simulink model "adm_pcie_9h7_dts_dual_4x100g_dsp_8b_1ant"  (R2019a)
settings: Solver=VariableStepAuto  StartTime=0.0  StopTime=10.0  RelTol=1e-3
undefined symbols (not defined in the file): datetime, fft_stages, posixtime
libraries: xbsIndex_r4 x17321, casper_library_misc x181, xps_library x11, casper_library_delays x8, casper_library_sources x8, casper_library_reorder x5, casper_library_scopes x4
(part 1 of 187)
settings Model: Creator=jackh  LastModifiedBy=mybur
settings Model: ModifiedComment=|
  | jackh -- Thu Feb 02 09:09:38 2023 -- Version 1.265
  | 
  | as compiled
settings Model: ModifiedHistory=|
  | jackh -- Thu Feb 02 09:09:38 2023 -- Version 1.265
  | 
  | as compiled
  | 
  | jackh -- Thu Feb 02 09:09:38 2023 -- Version 1.265
  | 
  | as compiled
  | 
  | jackh -- Wed Feb 01 20:29:00 2023 -- Version 1.264
  | 
  | Mitigate control change relating to 100G auto-shutoff which
  | prevents core from ever being manually disabled.
  | 
  | jackh -- Wed Jan 25 18:35:33 2023 -- Version 1.263
  | compiled 13.9
  | 
  | jackh -- Tue Jan 24 18:58:34 2023 -- Version 1.262
  | 
  | Increase non-fractional delay slope bits from 0 to 5,
  | allowing firmware-side delay extrapolation to run up to
  | 2^5 ADC samples
  | 
  | jackh -- Fri Jan 13 09:42:33 2023 -- Version 1.261
  | 
  | add options for DTS-error-induced auto 100G cutoff
  | 
  | jackh -- Thu Jan 12 13:56:07 2023 -- Version 1.260
  | 
  | Add automated 100GbE output halting on timing error detection
  | 
  | jackh -- Tue Nov 29 08:46:28 2022 -- Version 1.259
  | 
  | compiled
  | 
  | jackh -- Mon Nov 28 13:45:10 2022 -- Version 1.258
  | 
  | jackh -- Mon Nov 28 13:30:45 2022 -- Version 1.257
  | 
  | jackh -- Mon Nov 28 13:16:52 2022 -- Version 1.256
  | 
  | jackh -- Mon Nov 28 13:05:40 2022 -- Version 1.255
  | 
  | jackh -- Mon Nov 28 13:04:31 2022 -- Version 1.254
  | 
  | Bugfix -- negative fractional delays
  | 
  | jackh -- Wed Nov 23 08:43:33 2022 -- Version 1.253
  | 
  | as compiled
  | 
  | 
  | jackh -- Tue Nov 22 14:50:06 2022 -- Version 1.252
  | 
  | Rework LO precision.
  | - Make phase step register Fix45_44
  | - Allow periodic reloading
  | 
  | jackh -- Wed Nov 09 19:28:54 2022 -- Version 1.251
  | 
  | compiled
  | 
  | jackh -- Tue Nov 08 11:16:07 2022 -- Version 1.250
  | 
  | byteflip on pipeline 1 second 100G port
  | 
  | jackh -- Tue Nov 08 11:14:32 2022 -- Version 1.249
  | 
  | 13.7 -- dual 100G output
  | 
  | jackh -- Fri Nov 04 13:05:36 2022 -- Version 1.248
  | 
  | v13.7 -- use both 100G ports
  | 
  | jackh -- Mon Oct 10 10:09:12 2022 -- Version 1.247
  | 
  | as compiled
  | 
  | jackh -- Sun Oct 09 20:21:09 2022 -- Version 1.246
  | 
  | duplicate changes from LO shifter 0 for 1,2,3
  | 
  | jackh -- Sat Oct 08 20:23:11 2022 -- Version 1.245
  | as compiled
  | 
  | jackh -- Sat Oct 08 10:43:03 2022 -- Version 1.244
  | 
  | bugfix 2. Sync/data timing skew in phase rotate block
  | 
  | jackh -- Thu Oct 06 21:33:25 2022 -- Version 1.243
  | 
  | jackh -- Thu Oct 06 11:23:24 2022 -- Version 1.242
  | 
  | bugfix 1 -- timed sync in LO control should drive
  | reset of phase accumulators
  | 
  | jackh -- Thu Oct 06 10:04:46 2022 -- Version 1.241
  | 
  | compiled
  | 
  | jackh -- Wed Oct 05 14:02:44 2022 -- Version 1.240
  | 
  | v13.6
  | 
  | Add load time control for LO shift.
  | Use load time consistently through LO shift / coarse delay / phase rotate
  | 
  | jackh -- Wed Oct 05 08:55:34 2022 -- Version 1.239
  | 
  | compiled v13.5
  | 
  | jackh -- Tue Oct 04 17:52:52 2022 -- Version 1.238
  | 
  | v13.5
  | 
  | Make delay in delay tracking block signed
  | 
  | jackh -- Fri Sep 23 15:25:54 2022 -- Version 1.237
  | 
  | as compiled
  | 
  | jackh -- Thu Sep 22 10:47:01 2022 -- Version 1.236
  | 
  | Bugfix 5
  | Only allow syncs on TT multiples of 2^14 (probably 2^13 would
  | be sufficient -- this is the packetizer granularity)
  | Add reset logic to reorder (which has weird reorder-orders)
  | so that it only syncs off the first pulse after a reset
  | 
  | jackh -- Thu Sep 15 17:12:54 2022 -- Version 1.235
  | 
  | jackh -- Thu Sep 15 14:00:24 2022 -- Version 1.234
  | 
  | 13.4 bugfix 4 -- fix timing on TT load
  | 
  | jackh -- Wed Aug 24 08:02:53 2022 -- Version 1.233
  | 
  | compiled
  | 
  | jackh -- Tue Aug 23 14:04:43 2022 -- Version 1.232
  | 
  | v13.4 bugfix3 -- reduce data latency in DTS snapshot (cast) to balance sync
  | 
  | jackh -- Tue Aug 23 12:45:19 2022 -- Version 1.231
  | 
  | bugfix 2 -- recompile with oldest sample in DTS MSB.
  | Delay data relative to sync at DTS output so sync precedes by 1 clock
  | 
  | jackh -- Thu Aug 18 20:38:32 2022 -- Version 1.230
  | 
  | v13.4 bugfix 1
  | Rebuild with DTS buffer fixes
  | 
  | jackh -- Thu Aug 04 11:53:58 2022 -- Version 1.229
  | 
  | as compiled
  | 
  | jackh -- Wed Aug 03 18:39:00 2022 -- Version 1.228
  | 
  | v13.4 -- add post quant TVG which is a counter with spectrum number
  | 
  | jackh -- Wed Aug 03 12:22:54 2022 -- Version 1.227
  | 
  | as compiled
  | 
  | jackh -- Tue Aug 02 16:59:19 2022 -- Version 1.226
  | 
  | v13.3.3
  | 
  | Make LO offset input accept signed values
  | 
  | jackh -- Thu Jul 14 12:25:27 2022 -- Version 1.225
  | v13.3.2
  | 
  | change sine/cos lookup tables to 18-bit depth
  | 
  | jackh -- Fri Jul 08 12:09:48 2022 -- Version 1.224
  | 
  | jackh -- Fri Jul 08 11:59:21 2022 -- Version 1.223
  | 
  | 13.3.1
  | 
  | Make LO shift phase register 32_29
  | 
  | jackh -- Tue Jul 05 14:22:39 2022 -- Version 1.222
  | 
  | 13.2.4
  | 
  | Add 100G output snapshots and stats counters
  | 
  | jackh -- Fri Jun 17 09:21:46 2022 -- Version 1.221
  | 
  | Make PR template file relative. Increment fw revision
  | 
  | jackh -- Fri May 20 08:03:37 2022 -- Version 1.220
  | 
  | jackh -- Thu May 19 16:47:03 2022 -- Version 1.219
  | 
  | jackh -- Thu May 19 16:07:36 2022 -- Version 1.218
  | 
  | 13.2.2
  | 
  | Increase coarse delay to 512 samples
  | 
  | jackh -- Thu May 19 15:48:23 2022 -- Version 1.217
  | 
  | pipeline time offset
  | 
  | jackh -- Thu May 19 15:45:17 2022 -- Version 1.216
  | 
  | v13.2.1
  | 
  | Add aux time measurement
  | 
  | jackh -- Tue May 03 22:22:24 2022 -- Version 1.215
  | 
  | jackh -- Tue May 03 12:52:13 2022 -- Version 1.214
  | 
  | 13.2.0.1
  | 
  | - Fix FFT syncout period (now infinite)
  | - Add max_delay register to delay subsystem
  | 
  | jackh -- Tue May 03 11:06:51 2022 -- Version 1.213
  | 
  | v13.2 (should have been 13) as compiled
  | 
  | jackh -- Mon May 02 12:19:53 2022 -- Version 1.212
  | 
  | jackh -- Mon May 02 12:13:43 2022 -- Version 1.211
  | 
  | jackh -- Mon May 02 12:03:22 2022 -- Version 1.210
  | 
  | Move to 1MHz channels (2048-chan PFB; 1024 sent chans)
  | Incorporate FFT descramble mlib_devel fix
  | 
  | jackh -- Thu Apr 07 10:41:20 2022 -- Version 1.209
  | 
  | compiled
  | 
  | jackh -- Wed Apr 06 17:17:38 2022 -- Version 1.208
  | 
  | Bugfix 1
  | 
  | - Change LO offset so real part os cosine mixer (so mixing with DC does nothing)
  | - Fix cross-corr conjugation
  | - Fix cross corr acc_len computation
  | 
  | jackh -- Thu Mar 24 11:16:10 2022 -- Version 1.207
  | 
  | jackh -- Wed Mar 23 15:55:29 2022 -- Version 1.206
  | 
  | v12.2 Add sine wave generators to both pipelines.
  | Default to no added sine wave.
  | 
  | jackh -- Wed Mar 23 15:38:55 2022 -- Version 1.205
  | 
  | jackh -- Wed Mar 23 15:24:07 2022 -- Version 1.204
  | 
  | delay match sine generation and data streams
  | 
  | jackh -- Wed Mar 23 15:22:28 2022 -- Version 1.203
  | 
  | jackh -- Wed Mar 23 15:14:26 2022 -- Version 1.202
  | 
  | Add additive sinewave TVG
  | 
  | jackh -- Wed Mar 23 15:12:01 2022 -- Version 1.201
  | 
  | jackh -- Tue Mar 08 10:23:22 2022 -- Version 1.200
  | 
  | jackh -- Mon Mar 07 17:18:28 2022 -- Version 1.199
  | 
  | jackh -- Mon Mar 07 17:10:55 2022 -- Version 1.198
  | 
  | jackh -- Mon Mar 07 16:45:17 2022 -- Version 1.197
  | 
  | jackh -- Mon Mar 07 16:37:10 2022 -- Version 1.196
  | 
  | Add Corr block.
  | Allows examination of post-quantization signals, and
  | to cross correlate different IFs (useful for testing
  | in internal noisegen mode)
  | 
  | jackh -- Mon Mar 07 16:13:50 2022 -- Version 1.195
  | 
  | PFB band select reorder depth fix
  | 
  | jackh -- Thu Mar 03 13:08:01 2022 -- Version 1.194
  | 
  | jackh -- Tue Mar 01 20:34:16 2022 -- Version 1.193
  | 
  | jackh -- Tue Mar 01 17:19:43 2022 -- Version 1.192
  | 
  | jackh -- Tue Mar 01 17:10:04 2022 -- Version 1.191
  | 
  | jackh -- Tue Mar 01 16:55:54 2022 -- Version 1.190
  | 
  | jackh -- Tue Mar 01 16:45:57 2022 -- Version 1.189
  | 
  | jackh -- Tue Mar 01 15:57:56 2022 -- Version 1.188
  | 
  | jackh -- Tue Mar 01 15:49:45 2022 -- Version 1.187
  | 
  | jackh -- Tue Mar 01 15:22:14 2022 -- Version 1.186
  | 
  | jackh -- Mon Feb 28 13:26:19 2022 -- Version 1.185
  | 
  | jackh -- Mon Feb 28 13:08:19 2022 -- Version 1.184
  | 
  | jackh -- Sat Feb 26 14:41:54 2022 -- Version 1.183
  | 
  | jackh -- Fri Feb 25 18:46:11 2022 -- Version 1.182
  | 
  | jackh -- Fri Feb 25 18:45:03 2022 -- Version 1.181
  | 
  | jackh -- Thu Feb 24 15:51:36 2022 -- Version 1.180
  | 
  | update noisegen casting (just take MSBs)
  | 
  | jackh -- Thu Feb 24 15:08:58 2022 -- Version 1.179
  | 
  | v12
  | 
  | jackh -- Thu Feb 24 15:06:46 2022 -- Version 1.178
  | 
  | Move to 4x100G template
  | 
  | 
  | jackh -- Thu Feb 24 15:02:10 2022 -- Version 1.177
  | 
  | jackh -- Wed Feb 09 19:02:50 2022 -- Version 1.176
  | 
  | jackh -- Wed Feb 09 10:59:16 2022 -- Version 1.175
  | 
  | Try _again_ to fix timestamp issue.
  | This time the fix was actually simulated, and seems to work.
  | 
  | jackh -- Wed Feb 09 10:58:22 2022 -- Version 1.174
  | 
  | jackh -- Wed Feb 09 10:34:47 2022 -- Version 1.173
  | 
  | jackh -- Tue Feb 08 22:13:18 2022 -- Version 1.172
  | 
  | Change autocorr pipelining to fix timing errors
  | 
  | jackh -- Tue Feb 08 11:22:49 2022 -- Version 1.171
  | 
  | Try (again) to fix MCNT offset issue.
  | This time just propagate the time_step_bit lower MCNT counter
  | bits through to the header.
  | 
  | jackh -- Tue Feb 08 08:36:48 2022 -- Version 1.170
  | 
  | jackh -- Mon Feb 07 16:56:49 2022 -- Version 1.169
  | 
  | jackh -- Mon Feb 07 16:34:15 2022 -- Version 1.168
  | 
  | jackh -- Mon Feb 07 16:26:49 2022 -- Version 1.167
  | 
  | jackh -- Mon Feb 07 12:47:03 2022 -- Version 1.166
  | 
  | jackh -- Mon Feb 07 12:32:35 2022 -- Version 1.165
  | 
  | Add TT sync register, storing the time of the last sync
  | 
  | jackh -- Mon Feb 07 12:23:30 2022 -- Version 1.164
  | 
  | increment bugfix to 11.0.0.2
  | 
  | 
  | jackh -- Mon Feb 07 12:22:16 2022 -- Version 1.163
  | 
  | Propagate LSBs of sync time to packet headers
  | 
  | jackh -- Sat Feb 05 22:32:38 2022 -- Version 1.162
  | 
  | jackh -- Sat Feb 05 18:43:37 2022 -- Version 1.161
  | 
  | v11
  | More changes to reorder.
  | Process ADC data at 8 (not 12) bit resolution
  | Use URAM via black-box imports for coarse delay and big channel reorder
  | 
  | jackh -- Sat Feb 05 18:36:04 2022 -- Version 1.160
  | 
  | jackh -- Sat Feb 05 17:38:40 2022 -- Version 1.159
  | 
  | jackh -- Sat Feb 05 17:24:29 2022 -- Version 1.158
  | 
  | jackh -- Sat Feb 05 17:22:21 2022 -- Version 1.157
  | 
  | jackh -- Fri Feb 04 17:40:07 2022 -- Version 1.156
  | 
  | jackh -- Fri Feb 04 12:37:39 2022 -- Version 1.155
  | 
  | 64 times per packet
  | 
  | 
  | jackh -- Thu Feb 03 21:55:46 2022 -- Version 1.154
  | 
  | as compiled
  | 
  | 
  | jackh -- Thu Feb 03 14:45:04 2022 -- Version 1.153
  | 
  | jackh -- Thu Feb 03 14:28:02 2022 -- Version 1.152
  | 
  | jackh -- Thu Feb 03 13:59:18 2022 -- Version 1.151
  | 
  | jackh -- Thu Feb 03 11:15:21 2022 -- Version 1.150
  | 
  | jackh -- Wed Feb 02 16:47:47 2022 -- Version 1.149
  | 
  | jackh -- Wed Feb 02 16:40:11 2022 -- Version 1.148
  | 
  | Fix incorrect final transpose in reorder block
  | 
  | jackh -- Wed Feb 02 16:16:13 2022 -- Version 1.147
  | 
  | v8. Add channel reordering
  | 
  | Not actually necessary for 8-bit mode, but will
  | facilitate testing which is necessary for 3-bit mode
  | 
  | jackh -- Wed Feb 02 10:37:50 2022 -- Version 1.146
  | 
  | 7.0.1
  | 
  | Change coarse delay bram latency to 3 (hopefully will fix small timing fail)
  | 
  | jackh -- Wed Feb 02 10:34:03 2022 -- Version 1.145
  | 
  | jackh -- Tue Feb 01 14:52:02 2022 -- Version 1.144
  | 
  | Don't use ultraRAM for coarse delay (but we should!)
  | because it breaks sysgen. Sigh.
  | 
  | jackh -- Tue Feb 01 14:27:12 2022 -- Version 1.143
  | 
  | jackh -- Tue Feb 01 14:18:24 2022 -- Version 1.142
  | 
  | v7. Add noisegen / coarse delay
  | 
  | jackh -- Tue Feb 01 14:12:26 2022 -- Version 1.141
  | 
  | jackh -- Tue Feb 01 14:09:37 2022 -- Version 1.140
  | 
  | jackh -- Tue Feb 01 11:46:40 2022 -- Version 1.139
  | 
  | jackh -- Tue Feb 01 11:12:13 2022 -- Version 1.138
  | 
  | Add noise gen
  | 
  | jackh -- Tue Feb 01 11:01:17 2022 -- Version 1.137
  | 
  | v6.1 Harmonize input ordering convention by flipping
  | inputs so "input 0" is MSBs of data
  | 
  | jackh -- Tue Feb 01 10:38:57 2022 -- Version 1.136
  | 
  | jackh -- Mon Jan 31 13:11:04 2022 -- Version 1.135
  | 
  | jackh -- Mon Jan 31 12:33:38 2022 -- Version 1.134
  | 
  | jackh -- Mon Jan 31 12:25:15 2022 -- Version 1.133
  | 
  | jackh -- Fri Jan 28 17:22:49 2022 -- Version 1.132
  | 
  | jackh -- Fri Jan 28 17:16:19 2022 -- Version 1.131
  | 
  | jackh -- Fri Jan 28 17:06:25 2022 -- Version 1.130
  | 
  | v6.0 Add input bitstats / simulation mux
  | 
  | jackh -- Fri Jan 28 17:02:52 2022 -- Version 1.129
  | 
  | jackh -- Fri Jan 28 16:59:39 2022 -- Version 1.128
  | 
  | jackh -- Fri Jan 28 16:55:40 2022 -- Version 1.127
  | 
  | jackh -- Fri Jan 28 16:17:24 2022 -- Version 1.126
  | 
  | v5.0.2 Fix potential (but unliekly) issue with sync arm coinciding
  | with sync pulse
  | 
  | 
  | jackh -- Fri Jan 28 16:01:17 2022 -- Version 1.125
  | 
  | Attempt to fix DTS alignment unreliability (control signal CDC issue in mlib_devel)
  | 
  | jackh -- Fri Jan 28 12:51:42 2022 -- Version 1.124
  | 
  | as compiled
  | 
  | jackh -- Thu Jan 27 16:47:33 2022 -- Version 1.123
  | 
  | v5.0
  | 
  | Add sync gen logic
  | 
  | jackh -- Thu Jan 27 11:25:49 2022 -- Version 1.122
  | 
  | v4.1 Add index interval error counter
  | 
  | jackh -- Thu Jan 27 11:22:02 2022 -- Version 1.121
  | 
  | Make index 50ms -- add not-locked counter
  | 
  | 
  | jackh -- Thu Jan 27 10:32:00 2022 -- Version 1.120
  | 
  | Recompile using raw "index" pulse. Add index snapshots
  | 
  | jackh -- Wed Jan 26 15:06:47 2022 -- Version 1.119
  | 
  | jackh -- Wed Jan 26 13:46:28 2022 -- Version 1.118
  | 
  | jackh -- Wed Jan 26 13:04:56 2022 -- Version 1.117
  | 
  | jackh -- Tue Jan 25 18:32:15 2022 -- Version 1.116
  | 
  | Add index (10ms pulse?) count logic
  | 
  | jackh -- Tue Jan 25 18:31:36 2022 -- Version 1.115
  | 
  | jackh -- Tue Jan 25 11:48:12 2022 -- Version 1.114
  | 
  | jackh -- Tue Jan 25 11:41:44 2022 -- Version 1.113
  | 
  | jackh -- Tue Jan 25 11:38:37 2022 -- Version 1.112
  | 
  | Readd autocorr (needed behavioural complex mults)
  | 
  | jackh -- Mon Jan 24 20:49:54 2022 -- Version 1.111
  | 
  | comment out autocorr (causing compile fails)
  | 
  | jackh -- Mon Jan 24 20:10:36 2022 -- Version 1.110
  | 
  | jackh -- Mon Jan 24 19:58:33 2022 -- Version 1.109
  | 
  | jackh -- Mon Jan 24 19:53:28 2022 -- Version 1.108
  | 
  | autocorr floating point error fixes
  | 
  | 
  | jackh -- Mon Jan 24 19:51:34 2022 -- Version 1.107
  | 
  | jackh -- Mon Jan 24 18:28:31 2022 -- Version 1.106
  | 
  | jackh -- Mon Jan 24 18:27:12 2022 -- Version 1.105
  | 
  | Add autocorr (to pipeline 0)
  | 
  | jackh -- Mon Jan 24 18:15:24 2022 -- Version 1.104
  | 
  | Add EQTVG
  | 
  | jackh -- Mon Jan 24 13:19:54 2022 -- Version 1.103
settings DataIOCC: ReturnWorkspaceOutputs=off
settings DebuggingCC: PregeneratedLibrarySubsystemCodeDiagnostic=none  ArithmeticOperatorsInVariantConditions=warning
settings SFSimCC: SimUseLocalCustomCode=off
settings RTWCC: RTWUseLocalCustomCode=off

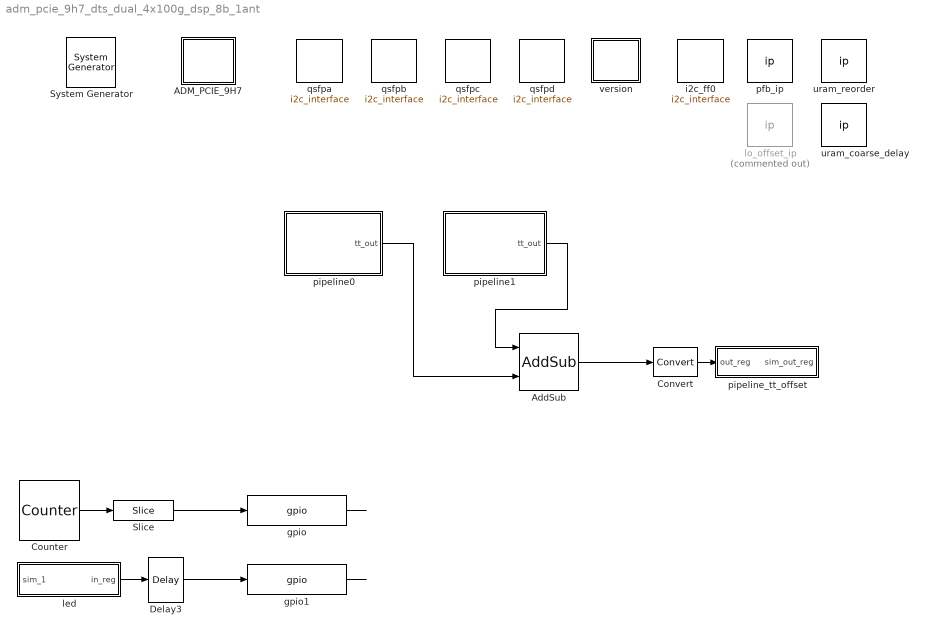
== system adm_pcie_9h7_dts_dual_4x100g_dsp_8b_1ant ==
  " System Generator" : xbsIndex_r4/ System Generator  Tag=genX  xilinxfamily=virtexuplusHBM  part=xcvu37p  speed=-2-e  package=fsvh2892  synthesis_tool=XST  clock_wrapper=Clock Enables  directory=/home/jackh/src/vla-dev/firmware/adm_pcie_9h7_dts_dual_4x100g_dsp_8b/sysgen  proj_type=Vivado  Synth_file=Vivado Synthesis Defaults  Impl_file=Vivado Implementation Defaults  testbench=off  simulink_period=1  sysclk_period=3.9062  dcm_input_clock_period=10  incr_netlist=off  trim_vbits=Everywhere in SubSystem  dbl_ovrd=According to Block Masks  core_generation=According to Block Masks  run_coregen=off  deprecated_control=off  eval_field=0  block_type=sysgen
  ADM_PCIE_9H7 : Subsystem  Tag=xps:xsg  mask(xsg core config){hw_sys=ADM_PCIE_9H7:xcvu37p, clk_src=dts_clk, clk_rate=256, use_microblaze=off, use_pr=on, pr_template=[fileparts(which(bdroot)) '/pr_templates/adm_pcie_9h7_dts_dual_4x100g_pr_template-no-ip.xpr.zip'], sample_period=1, synthesis_tool=XST}
      mask prompts: hw_sys "Hardware Platform"; clk_src "User IP Clock source"; clk_rate "User IP Clock Rate (MHz)"; use_microblaze "Use Microblaze controller?"; use_pr "Use PCIe Partial Reconfiguration"; sample_period "Sample Period"; synthesis_tool "Synthesis Tool:"
      mask help:
      | The XSG Core Config block is used to configure the System Generator design
      | for the casper_xps toolflow. Settings here are used to configure the
      | Xilinx System Generator block parameters automatically, and control toolflow
      | script  execution. It needs to be at the top level of all designs being compiled
      | with the casper_xps toolflow.
      mask init:
      | xps_xsg_adm_pcie_9h7_conf_mask;
      mask Help: eval('xlWeb([getenv(''MLIB_ROOT''), ''\doc\html\sys_xsg_core_config\sys_xsg_core_config.html''])')
      mask TypeOptions hw_sys: ADM_PCIE_9H7:xcvu37p
      mask TypeOptions clk_src: sys_clk | dts_clk
      mask TypeOptions synthesis_tool: Leonardo Spectrum | Synplify | Synplify Pro | XST
      mask Display: fprintf(['ADM\nPCIE_9H7']);
  AddSub : xbsIndex_r4/AddSub  mode=Subtraction  use_carryin=off  use_carryout=off  en=off  latency=3  precision=Full  arith_type=Unsigned  n_bits=16  bin_pt=14  quantization=Truncate  overflow=Wrap  use_behavioral_HDL=off  hw_selection=Fabric  pipelined=on  dbl_ovrd=off  block_type=addsub
  Convert : xbsIndex_r4/Convert  gui_display_data_type=Fixed-point  arith_type="Signed  (2's comp)"  n_bits=32  bin_pt=0  float_type=Single  exp_bits=8  fraction_bits=24  quantization=Truncate  overflow=Wrap  en=off  latency=1  pipeline=off  dbl_ovrd=off  block_type=convert
  Counter : xbsIndex_r4/Counter  cnt_type=Free Running  cnt_to=Inf  operation=Up  start_count=0  cnt_by_val=1  arith_type=Unsigned  n_bits=27  bin_pt=0  load_pin=off  rst=off  en=off  explicit_period=on  period=1  use_behavioral_HDL=off  implementation=Fabric  dbl_ovrd=off  block_type=counter
  Delay3 : xbsIndex_r4/Delay  rst=off  infoeditControl=Selection of Reset will increase slice count due to use of real FFs and instead of SRLs  en=off  latency=1  reg_retiming=off  dbl_ovrd=off  block_type=delay
  Slice : xbsIndex_r4/Slice  nbits=2  boolean_output=off  mode=Upper Bit Location + Width  bit1=0  base1=MSB of Input  bit0=0  base0=LSB of Input  dbl_ovrd=off  block_type=slice
  gpio : xps_library/IO/gpio  Tag=xps:gpio  io_group_params_forwarded=off  io_group=ROACH:led  io_group_real=led  io_group_custom=0  io_dir=out  arith_type=Unsigned  bitwidth=2  bin_pt=0  bit_index=[0 1]  sample_period=1  use_single_ended=off  use_ddr=off  reg_iob=on  reg_clk_phase=0  termination=None
      settings: SourceProductName=CASPER XPS Blockset
  gpio1 : xps_library/IO/gpio  Tag=xps:gpio  io_group_params_forwarded=off  io_group=ROACH:led  io_group_real=led  io_group_custom=0  io_dir=out  arith_type=Boolean  bitwidth=1  bin_pt=0  bit_index=2  sample_period=1  use_single_ended=off  use_ddr=off  reg_iob=on  reg_clk_phase=0  termination=None
      settings: SourceProductName=CASPER XPS Blockset
  i2c_ff0 : xps_library/IO/i2c_interface  Tag=xps:i2c_interface  sda_gpio='gpio'  sda_gpio_index=8  scl_gpio='gpio'  scl_gpio_index=7
      settings: SourceProductName=CASPER XPS Blockset
  led : Subsystem  Tag=xps:sw_reg  AncestorBlock=xps_library/Memory/software_register  mask(swreg){io_dir=From Processor, io_delay=0, init_val=0, sample_period=1, names=reg, bitwidths=1, bin_pts=0, arith_types=2, sim_port=on, show_format=on}
      mask prompts: io_dir "I/O direction"; io_delay "I/O delay"; init_val "Initial Value"; sample_period "Sample period"; names "Bitfield names [msb...lsb]"; bitwidths "Bitfield widths"; bin_pts "Bitfield binary pts"; arith_types "Bitfield types, ufix=0, fix=1, bool=2"; sim_port "Provide sim input/output?"; show_format "Print format string?"
      mask help: A 32-bit software-accessible register. Can be divided into bitfields of varying widths and types using the fields in the block mask.
      mask init:
      | swreg_init(gcb)
      settings: AttributesFormatString=1input:b = 1 bits
      mask TypeOptions io_dir: To Processor | From Processor
      mask Callback io_dir:
      | mask_enables = get_param(gcb, 'MaskEnables');
      | mask_names = get_param(gcb, 'MaskNames');
      | if strcmp(get_param(gcb, 'io_dir'), 'To Processor'),
      |     mask_enables{ismember(mask_names, 'sample_period')} = 'off';
      | else
      |     mask_enables{ismember(mask_names, 'sample_period')} = 'on';
      | end
      | set_param(gcb, 'MaskEnables', mask_enables);
      mask DialogControl ParameterTabVar0 Prompt: Setup
  lo_offset_ip : xps_library/Utilities/ip  Tag=xps:ip  Commented=on  lib_path=[fileparts(which(bdroot)) '/dsp/mixer_dec_8x_8i_8o_core']  ip_name='mixer_dec_8x_8i_8o_core'
      settings: SourceProductName=CASPER XPS Blockset
  pfb_ip : xps_library/Utilities/ip  Tag=xps:ip  lib_path=[fileparts(which(bdroot)) '/dsp/pfb_cplx_2p_2048c_16i_18o_core']  ip_name='pfb_cplx_2p_2048c_16i_18o_core'
      settings: SourceProductName=CASPER XPS Blockset
  pipeline0 : Subsystem
  pipeline1 : Subsystem
  pipeline_tt_offset : Subsystem  Tag=xps:sw_reg  AncestorBlock=xps_library/Memory/software_register  mask(swreg){io_dir=To Processor, io_delay=0, init_val=0, sample_period=1, names=reg, bitwidths=32, bin_pts=0, arith_types=1, sim_port=on, show_format=on}
      mask prompts: io_dir "I/O direction"; io_delay "I/O delay"; init_val "Initial Value"; sample_period "Sample period"; names "Bitfield names [msb...lsb]"; bitwidths "Bitfield widths"; bin_pts "Bitfield binary pts"; arith_types "Bitfield types, ufix=0, fix=1, bool=2"; sim_port "Provide sim input/output?"; show_format "Print format string?"
      mask help: A 32-bit software-accessible register. Can be divided into bitfields of varying widths and types using the fields in the block mask.
      mask init:
      | swreg_init(gcb)
      settings: AttributesFormatString=1output:f32.0 = 32 bits
      mask TypeOptions io_dir: To Processor | From Processor
      mask Callback io_dir:
      | mask_enables = get_param(gcb, 'MaskEnables');
      | mask_names = get_param(gcb, 'MaskNames');
      | if strcmp(get_param(gcb, 'io_dir'), 'To Processor'),
      |     mask_enables{ismember(mask_names, 'sample_period')} = 'off';
      | else
      |     mask_enables{ismember(mask_names, 'sample_period')} = 'on';
      | end
      | set_param(gcb, 'MaskEnables', mask_enables);
      mask DialogControl ParameterTabVar0 Prompt: Setup
  qsfpa : xps_library/IO/i2c_interface  Tag=xps:i2c_interface  sda_gpio='qsfp_sda'  sda_gpio_index=0  scl_gpio='qsfp_scl'  scl_gpio_index=0
      settings: SourceProductName=CASPER XPS Blockset
  qsfpb : xps_library/IO/i2c_interface  Tag=xps:i2c_interface  sda_gpio='qsfp_sda'  sda_gpio_index=1  scl_gpio='qsfp_scl'  scl_gpio_index=1
      settings: SourceProductName=CASPER XPS Blockset
  qsfpc : xps_library/IO/i2c_interface  Tag=xps:i2c_interface  sda_gpio='qsfp_sda'  sda_gpio_index=2  scl_gpio='qsfp_scl'  scl_gpio_index=2
      settings: SourceProductName=CASPER XPS Blockset
  qsfpd : xps_library/IO/i2c_interface  Tag=xps:i2c_interface  sda_gpio='qsfp_sda'  sda_gpio_index=3  scl_gpio='qsfp_scl'  scl_gpio_index=3
      settings: SourceProductName=CASPER XPS Blockset
  uram_coarse_delay : xps_library/Utilities/ip  Tag=xps:ip  lib_path=[fileparts(which(bdroot)) '/dsp/uram_dp_64kx64_latency3_core']  ip_name='uram_dp_64kx64_latency3_core'
      settings: SourceProductName=CASPER XPS Blockset
  uram_reorder : xps_library/Utilities/ip  Tag=xps:ip  lib_path=[fileparts(which(bdroot)) '/dsp/uram_8192x512_latency3_core']  ip_name='uram_8192x512_latency3_core'
      settings: SourceProductName=CASPER XPS Blockset
  version : Subsystem  mask{fw_type=4, ver_maj=13, ver_min=9, ver_rev=0, ver_bugfix=1}
      mask prompts: fw_type "Firmware Type"; ver_maj "Major version"; ver_min "Minor version"; ver_rev "Revision"; ver_bugfix "Bugfix"
  wires:
  gpio/1 -> ?
  Delay3/1 -> gpio1/1
  Counter/1 -> Slice/1
  gpio1/1 -> ?
  led/1(in_reg) -> Delay3/1
  Slice/1 -> gpio/1
  pipeline1/1(tt_out) -> AddSub/1
  pipeline0/1(tt_out) -> AddSub/2
  AddSub/1 -> Convert/1
  Convert/1 -> pipeline_tt_offset/1(out_reg)

== system adm_pcie_9h7_dts_dual_4x100g_dsp_8b_1ant/ADM_PCIE_9H7 ==

== system adm_pcie_9h7_dts_dual_4x100g_dsp_8b_1ant/led ==
  sim_1 : Inport
  adm_pcie_9h7_dts_dual_4x100g_dsp_8b_1ant_led_user_data_out : xbsIndex_r4/Gateway In  gui_display_data_type=Fixed-point  arith_type=Unsigned  n_bits=32  bin_pt=0  preci_type=Single  exp_width=8  frac_width=24  rows=1  columns=1  quantization="Round  (unbiased: +/- Inf)"  overflow=Saturate  period=1  UseAsADC=off  ADCChannel='1'  interface=None  automatic_assignment=on  address_offset=hex2dec('00')  intf_name=''  intf_description=''  default_value=0  timing_constraint=None  locs_specified=off  LOCs={}  io_standard={}  inherit_from_input=off  hdl_port=on  dbl_ovrd=off  block_type=gatewayin
  convert1_1 : DataTypeConversion  OutDataTypeStr=fixdt('ufix1_En0')  LockScale=on
  convert2_1 : DataTypeConversion  OutDataTypeStr=fixdt('ufix1_En0')  ConvertRealWorld=Stored Integer (SI)  LockScale=on
  gain_1 : Gain
  io_delay : xbsIndex_r4/Delay  rst=off  infoeditControl=Selection of Reset will increase slice count due to use of real FFs and instead of SRLs  en=off  latency=0  reg_retiming=on  dbl_ovrd=off  block_type=delay
  slice_reg : xbsIndex_r4/Slice  nbits=1  boolean_output=on  mode=Lower Bit Location + Width  bit1=0  base1=MSB of Input  bit0=0  base0=LSB of Input  dbl_ovrd=off  block_type=slice
  in_reg : Outport
  wires:
  adm_pcie_9h7_dts_dual_4x100g_dsp_8b_1ant_led_user_data_out/1 -> io_delay/1
  sim_1/1 -> convert1_1/1
  convert1_1/1 -> convert2_1/1
  convert2_1/1 -> gain_1/1
  gain_1/1 -> adm_pcie_9h7_dts_dual_4x100g_dsp_8b_1ant_led_user_data_out/1
  io_delay/1 -> slice_reg/1
  slice_reg/1 -> in_reg/1

== system adm_pcie_9h7_dts_dual_4x100g_dsp_8b_1ant/pipeline0 ==
  note: 4 inputs (2 IFs x dual pol)
      |
      | Each 8 parallel words x 12 bits
      | (96 bits per input)
      | (384 bits total)
  autocorr : Subsystem  mask{nchan_bits=10-2, npol_bits=0}
      mask prompts: nchan_bits "Number of *SERIAL* channels (2^?)"; npol_bits "Number of pols (2^?)"
  bus_convert1 : Subsystem  AncestorBlock=casper_library_bus/bus_convert  mask(bus_convert){n_bits_in=12*ones(4*8,1), bin_pt_in=11, cmplx=off, n_bits_out=8, bin_pt_out=7, quantization=0, overflow=0, csp_latency=0, of=off, misc=off}
      mask prompts: n_bits_in "input bit widths"; bin_pt_in "input binary points"; cmplx "input complex"; n_bits_out "output bit widths"; bin_pt_out "output binary points"; quantization "quantization strategy (Truncate=0, Round  (unbiased: +/- Inf)=1, Round (unbiased: Even Values)=2)"; overflow "overflow strategy (Wrap=0, Saturate=1, Flag as error=2)"; csp_latency "latency"; of "overflow indication"; misc "misc support"
      mask help: Convert components of busses
      mask init:
      | bus_convert_init(gcb, ...
      |     'n_bits_in', n_bits_in, ...
      |     'bin_pt_in', bin_pt_in, ...
      |     'cmplx', cmplx, ...
      |     'n_bits_out', n_bits_out, ...
      |     'bin_pt_out', bin_pt_out, ...
      |     'quantization', quantization, ...
      |     'overflow', overflow, ...
      |     'csp_latency', csp_latency, ...
      |     'misc', misc, ...
      |     'of', of);
  byte_flip : Subsystem  AncestorBlock=casper_library_flow_control/munge  mask(munge){divisions=64, div_size=8*ones(1,64), order=[63:-1:0], arith_type_out=Unsigned, bin_pt_out=0}
      mask prompts: divisions "Number of divisions"; div_size "Division size (bits)"; order "Division packing order"; arith_type_out "Output arithmetic type"; bin_pt_out "Output binary point"
      mask help: Splits an input bus into the specified number of divisions and then recombines them in the order specified (most significant division = 0,least = number divisions-1)
      mask init:
      | munge_init(gcb, ...
      |     'divisions', divisions, ...
      |     'div_size', div_size, ...
      |     'order', order, ...
      |     'arith_type_out', arith_type_out, ...
      |     'bin_pt_out', bin_pt_out);
      settings: AttributesFormatString=|
      | split:[8 8 8 8 8 8 8 8 8 8 8 8 8 8 8 8 8 8 8 8 8 8 8 8 8 8 8 8 8 8 8 8 8 8 8 8 8 8 8 8 8 8 8 8 8 8 8 8 8 8 8 8 8 8 8 8 8 8 8 8 8 8 8 8]
      | join:[63 62 61 60 59 58 57 56 55 54 53 52 51 50 49 48 47 46 45 44 43 42 41 40 39 38 37 36 35 34 33 32 31 30 29 28 27 26 25 24 23 22 21 20 19 18 17 16 15 14 13 12 11 10 9 8 7 6 5 4 3 2 1 0]
      | Unsigned [512,0]
      mask TypeOptions arith_type_out: Unsigned | Signed  (2's comp) | Floating-point
  byte_flip1 : Subsystem  AncestorBlock=casper_library_flow_control/munge  mask(munge){divisions=64, div_size=8*ones(1,64), order=[63:-1:0], arith_type_out=Unsigned, bin_pt_out=0}
      mask prompts: divisions "Number of divisions"; div_size "Division size (bits)"; order "Division packing order"; arith_type_out "Output arithmetic type"; bin_pt_out "Output binary point"
      mask help: Splits an input bus into the specified number of divisions and then recombines them in the order specified (most significant division = 0,least = number divisions-1)
      mask init:
      | munge_init(gcb, ...
      |     'divisions', divisions, ...
      |     'div_size', div_size, ...
      |     'order', order, ...
      |     'arith_type_out', arith_type_out, ...
      |     'bin_pt_out', bin_pt_out);
      settings: AttributesFormatString=|
      | split:[8 8 8 8 8 8 8 8 8 8 8 8 8 8 8 8 8 8 8 8 8 8 8 8 8 8 8 8 8 8 8 8 8 8 8 8 8 8 8 8 8 8 8 8 8 8 8 8 8 8 8 8 8 8 8 8 8 8 8 8 8 8 8 8]
      | join:[63 62 61 60 59 58 57 56 55 54 53 52 51 50 49 48 47 46 45 44 43 42 41 40 39 38 37 36 35 34 33 32 31 30 29 28 27 26 25 24 23 22 21 20 19 18 17 16 15 14 13 12 11 10 9 8 7 6 5 4 3 2 1 0]
      | Unsigned [512,0]
      mask TypeOptions arith_type_out: Unsigned | Signed  (2's comp) | Floating-point
  corr : Subsystem  mask{nchan_serial_bits=10-2}
      mask prompts: nchan_serial_bits "Number of serial channels (2^?)"
  delay : Subsystem
  dts : Subsystem
  eq : Subsystem
  eth0 : Subsystem
  eth1 : Subsystem
  input : Subsystem
  lo : Subsystem
  noise : Subsystem
  offset1 : Subsystem
  packetizer0 : Subsystem  mask{nchan_bits=10, npol_bits=(2+1)+5, nparallel_bits=5, step_bits=2, time_step_bits=5}
      mask prompts: nchan_bits "Number of channels (including unsent) (2^?)"; npol_bits "Number of pols*times (2^?)"; nparallel_bits "Parallel samples (2^?) Single-pol, single-chan, single-time samples per parallel word"; step_bits "Step (packet) granularity (2^?)"; time_step_bits "Time Steps per cycle (2^?). This is the amount the packet index is incremented by with each full sending cycle."
  packetizer1 : Subsystem  mask{nchan_bits=10, npol_bits=(2+1)+5, nparallel_bits=5, step_bits=2, time_step_bits=5}
      mask prompts: nchan_bits "Number of channels (including unsent) (2^?)"; npol_bits "Number of pols*times (2^?)"; nparallel_bits "Parallel samples (2^?) Single-pol, single-chan, single-time samples per parallel word"; step_bits "Step (packet) granularity (2^?)"; time_step_bits "Time Steps per cycle (2^?). This is the amount the packet index is incremented by with each full sending cycle."
  pfb : Subsystem
  phase_rotate : Subsystem  mask{in_bits=18, n_chan_bits=10}
      mask prompts: in_bits "Data in bitwidth (per word)"; n_chan_bits "Number of frequency channels (2^?)"
  post_eq_tvg : Subsystem  mask{chan_bits=10, parallel_bits=2}
      mask prompts: chan_bits "Frequency Channels (2^?)"; parallel_bits "Parallel samples (2^?)"
  reorder : Subsystem
  sine_tvg : Subsystem
  sync : Subsystem  mask{sync_lsb_bits=14, sync_period=12800000}
      mask prompts: sync_lsb_bits "Allowed sync granularity (2^?)"; sync_period "Expected_sync_period"
  two_comp : Subsystem
  tt_out : Outport
  wires:
  offset1/1(dout) -> packetizer1/2(data_in), packetizer0/2(data_in)
  reorder/1(sync_out) -> packetizer1/1(sync_in), packetizer0/1(sync_in)
  reorder/2(dout) -> offset1/1(din)
  packetizer0/1(data_out) -> byte_flip/1(din)
  packetizer0/3(eof) -> eth0/3(eof)
  packetizer0/4(dest_ip) -> eth0/4(dest_ip)
  packetizer0/5(dest_port) -> eth0/5(dest_port)
  packetizer0/6(byte_enable) -> eth0/6(byte_enable)
  byte_flip/1(dout) -> eth0/1(data)
  packetizer0/2(valid_out) -> eth0/2(vld)
  phase_rotate/1(sync_out) -> eq/1(sync)
  phase_rotate/2(dout) -> eq/2(din)
  pfb/1(sync_out) -> phase_rotate/1(sync), autocorr/1(sync)
  pfb/2(dout) -> phase_rotate/2(din), autocorr/2(din)
  [mrst] -> phase_rotate/3(mrst)
  eq/1(sync_out) -> post_eq_tvg/1(sync)
  eq/2(dout) -> post_eq_tvg/2(din)
  post_eq_tvg/1(sync_out) -> corr/1(sync), reorder/1(sync)
  post_eq_tvg/2(dout) -> corr/2(din), reorder/2(din)
  [mrst] -> autocorr/3(rst)
  sync/3(ext_sync) -> [sync_trig]
  sync/2(tt_sync) -> [sync_time]
  sync/4(sync_out) -> [sync_gen]
  sync/1(arm_noise) -> [arm_noise]
  sync/5(mrst) -> [mrst]
  sync/6(adc_sync) -> [adc_sync]
  dts/1(sync) -> sync/1(sync_in)
  [mrst] -> packetizer0/3(mrst_in)
  [ver_maj] -> packetizer0/4(version)
  [sync_time] -> packetizer0/5(sync_time)
  [sync_gen] -> input/3(sync)
  dts/2(dout) -> two_comp/1(In1)
  [sync_gen] -> noise/1(sync_in)
  [arm_noise] -> noise/2(arm_noise)
  noise/1(noise) -> input/2(noise)
  bus_convert1/1(dout) -> input/1(adc)
  two_comp/1(Out1) -> bus_convert1/1(din)
  [mrst] -> delay/3(mrst)
  [sync_time] -> delay/4(sync_time)
  delay/1(sync_out) -> lo/1(sync)
  delay/2(dout) -> lo/2(din)
  [mrst] -> lo/3(rst)
  lo/1(sync_out) -> pfb/1(sync)
  lo/2(dout) -> pfb/2(din)
  input/1(sync_out) -> sine_tvg/1(sync)
  input/2(dout) -> sine_tvg/2(din)
  sine_tvg/1(sync_out) -> delay/1(sync)
  sine_tvg/2(dout) -> delay/2(din)
  sync/7(tt_int_out) -> tt_out/1
  [mrst] -> reorder/3(mrst_in)
  [sync_time] -> phase_rotate/4(sync_time)
  [sync_time] -> lo/4(sync_time)
  packetizer1/2(valid_out) -> eth1/2(vld)
  byte_flip1/1(dout) -> eth1/1(data)
  packetizer1/6(byte_enable) -> eth1/6(byte_enable)
  packetizer1/5(dest_port) -> eth1/5(dest_port)
  packetizer1/4(dest_ip) -> eth1/4(dest_ip)
  packetizer1/3(eof) -> eth1/3(eof)
  packetizer1/1(data_out) -> byte_flip1/1(din)
  [mrst] -> packetizer1/3(mrst_in)
  [ver_maj] -> packetizer1/4(version)
  [sync_time] -> packetizer1/5(sync_time)
  sync/8(err_out) -> [time_error]
  [time_error] -> eth0/7(halt)
  [time_error] -> eth1/7(halt)

== system adm_pcie_9h7_dts_dual_4x100g_dsp_8b_1ant/pipeline1 ==
  note: 4 inputs (2 IFs x dual pol)
      |
      | Each 8 parallel words x 12 bits
      | (96 bits per input)
      | (384 bits total)
  note: SINGLE-ANTENNA 8-BIT BUILD (fw_type=4).
      | pipeline1 DSP removed. DTS and 2x 100GbE kept: the PR shell requires 2 DTS + 4 eth.
      | eth0/eth1 tx inputs tied to zero (never transmit). Antenna must use pipeline0 DTS (qsfp_a_b_c, clock master).
  dts : Subsystem
  dts_dout_term : Terminator
  eth0 : Subsystem
  eth0_byte_enable_zero : xbsIndex_r4/Constant  const=0  gui_display_data_type=Fixed-point  arith_type=Unsigned  n_bits=64  bin_pt=0  preci_type=Single  exp_width=8  frac_width=24  explicit_period=on  period=1  equ=P=C  opselect=C  inp2=PCIN>>17  opr=+  inp1=P  carry=CIN  dbl_ovrd=off  block_type=constant
  eth0_data_zero : xbsIndex_r4/Constant  const=0  gui_display_data_type=Fixed-point  arith_type=Unsigned  n_bits=512  bin_pt=0  preci_type=Single  exp_width=8  frac_width=24  explicit_period=on  period=1  equ=P=C  opselect=C  inp2=PCIN>>17  opr=+  inp1=P  carry=CIN  dbl_ovrd=off  block_type=constant
  eth0_dest_ip_zero : xbsIndex_r4/Constant  const=0  gui_display_data_type=Fixed-point  arith_type=Unsigned  n_bits=32  bin_pt=0  preci_type=Single  exp_width=8  frac_width=24  explicit_period=on  period=1  equ=P=C  opselect=C  inp2=PCIN>>17  opr=+  inp1=P  carry=CIN  dbl_ovrd=off  block_type=constant
  eth0_dest_port_zero : xbsIndex_r4/Constant  const=0  gui_display_data_type=Fixed-point  arith_type=Unsigned  n_bits=16  bin_pt=0  preci_type=Single  exp_width=8  frac_width=24  explicit_period=on  period=1  equ=P=C  opselect=C  inp2=PCIN>>17  opr=+  inp1=P  carry=CIN  dbl_ovrd=off  block_type=constant
  eth0_eof_zero : xbsIndex_r4/Constant  const=0  gui_display_data_type=Fixed-point  arith_type=Boolean  n_bits=1  bin_pt=0  preci_type=Single  exp_width=8  frac_width=24  explicit_period=on  period=1  equ=P=C  opselect=C  inp2=PCIN>>17  opr=+  inp1=P  carry=CIN  dbl_ovrd=off  block_type=constant
  eth0_vld_zero : xbsIndex_r4/Constant  const=0  gui_display_data_type=Fixed-point  arith_type=Boolean  n_bits=1  bin_pt=0  preci_type=Single  exp_width=8  frac_width=24  explicit_period=on  period=1  equ=P=C  opselect=C  inp2=PCIN>>17  opr=+  inp1=P  carry=CIN  dbl_ovrd=off  block_type=constant
  eth1 : Subsystem
  eth1_byte_enable_zero : xbsIndex_r4/Constant  const=0  gui_display_data_type=Fixed-point  arith_type=Unsigned  n_bits=64  bin_pt=0  preci_type=Single  exp_width=8  frac_width=24  explicit_period=on  period=1  equ=P=C  opselect=C  inp2=PCIN>>17  opr=+  inp1=P  carry=CIN  dbl_ovrd=off  block_type=constant
  eth1_data_zero : xbsIndex_r4/Constant  const=0  gui_display_data_type=Fixed-point  arith_type=Unsigned  n_bits=512  bin_pt=0  preci_type=Single  exp_width=8  frac_width=24  explicit_period=on  period=1  equ=P=C  opselect=C  inp2=PCIN>>17  opr=+  inp1=P  carry=CIN  dbl_ovrd=off  block_type=constant
  eth1_dest_ip_zero : xbsIndex_r4/Constant  const=0  gui_display_data_type=Fixed-point  arith_type=Unsigned  n_bits=32  bin_pt=0  preci_type=Single  exp_width=8  frac_width=24  explicit_period=on  period=1  equ=P=C  opselect=C  inp2=PCIN>>17  opr=+  inp1=P  carry=CIN  dbl_ovrd=off  block_type=constant
  eth1_dest_port_zero : xbsIndex_r4/Constant  const=0  gui_display_data_type=Fixed-point  arith_type=Unsigned  n_bits=16  bin_pt=0  preci_type=Single  exp_width=8  frac_width=24  explicit_period=on  period=1  equ=P=C  opselect=C  inp2=PCIN>>17  opr=+  inp1=P  carry=CIN  dbl_ovrd=off  block_type=constant
  eth1_eof_zero : xbsIndex_r4/Constant  const=0  gui_display_data_type=Fixed-point  arith_type=Boolean  n_bits=1  bin_pt=0  preci_type=Single  exp_width=8  frac_width=24  explicit_period=on  period=1  equ=P=C  opselect=C  inp2=PCIN>>17  opr=+  inp1=P  carry=CIN  dbl_ovrd=off  block_type=constant
  eth1_vld_zero : xbsIndex_r4/Constant  const=0  gui_display_data_type=Fixed-point  arith_type=Boolean  n_bits=1  bin_pt=0  preci_type=Single  exp_width=8  frac_width=24  explicit_period=on  period=1  equ=P=C  opselect=C  inp2=PCIN>>17  opr=+  inp1=P  carry=CIN  dbl_ovrd=off  block_type=constant
  sync : Subsystem  mask{sync_lsb_bits=14, sync_period=12800000}
      mask prompts: sync_lsb_bits "Allowed sync granularity (2^?)"; sync_period "Expected_sync_period"
  tt_out : Outport
  wires:
  dts/1(sync) -> sync/1(sync_in)
  sync/3(ext_sync) -> [sync_trig]
  sync/5(mrst) -> [mrst]
  sync/2(tt_sync) -> [sync_time]
  sync/8(err_out) -> [time_error]
  sync/7(tt_int_out) -> tt_out/1
  sync/6(adc_sync) -> [adc_sync]
  sync/1(arm_noise) -> [arm_noise]
  sync/4(sync_out) -> [sync_gen]
  [time_error] -> eth0/7(halt)
  [time_error] -> eth1/7(halt)
  eth0_data_zero/1 -> eth0/1(data)
  eth0_vld_zero/1 -> eth0/2(vld)
  eth0_eof_zero/1 -> eth0/3(eof)
  eth0_dest_ip_zero/1 -> eth0/4(dest_ip)
  eth0_dest_port_zero/1 -> eth0/5(dest_port)
  eth0_byte_enable_zero/1 -> eth0/6(byte_enable)
  eth1_data_zero/1 -> eth1/1(data)
  eth1_vld_zero/1 -> eth1/2(vld)
  eth1_eof_zero/1 -> eth1/3(eof)
  eth1_dest_ip_zero/1 -> eth1/4(dest_ip)
  eth1_dest_port_zero/1 -> eth1/5(dest_port)
  eth1_byte_enable_zero/1 -> eth1/6(byte_enable)
  dts/2(dout) -> dts_dout_term/1

== system adm_pcie_9h7_dts_dual_4x100g_dsp_8b_1ant/pipeline_tt_offset ==
  out_reg : Inport
  adm_pcie_9h7_dts_dual_4x100g_dsp_8b_1ant_pipeline_tt_offset_user_data_in : xbsIndex_r4/Gateway Out  inherit_from_input=off  hdl_port=on  rows=1  columns=1  UseAsDAC=off  DACChannel='1'  interface=None  automatic_assignment=on  address_offset=hex2dec('00')  intf_name=''  intf_description=''  timing_constraint=None  locs_specified=off  LOCs={}  io_standard={}  block_type=gatewayout
  assert_reg : xbsIndex_r4/Assert  assert_type=on  type_source=Explicitly  gui_display_data_type=Fixed-point  arith_type="Signed  (2's comp)"  n_bits=32  bin_pt=0  preci_type=Single  exp_width=8  frac_width=24  assert_rate=off  rate_source=Explicitly  period=1  output_port=on  block_type=assert
  cast_gw : xbsIndex_r4/Convert  gui_display_data_type=Fixed-point  arith_type=Unsigned  n_bits=32  bin_pt=0  float_type=Single  exp_bits=8  fraction_bits=24  quantization=Truncate  overflow=Wrap  en=off  latency=1  pipeline=off  dbl_ovrd=off  block_type=convert
  io_delay : xbsIndex_r4/Delay  rst=off  infoeditControl=Selection of Reset will increase slice count due to use of real FFs and instead of SRLs  en=off  latency=0  reg_retiming=on  dbl_ovrd=off  block_type=delay
  reint1 : xbsIndex_r4/Reinterpret  force_arith_type=on  arith_type=Unsigned  force_bin_pt=on  bin_pt=0  block_type=reinterpret
  sim_out : Terminator
  sim_out_reg_gw : xbsIndex_r4/Gateway Out  inherit_from_input=off  hdl_port=off  rows=1  columns=1  UseAsDAC=off  DACChannel='1'  interface=None  automatic_assignment=on  address_offset=hex2dec('00')  intf_name=''  intf_description=''  timing_constraint=None  locs_specified=off  LOCs={}  io_standard={}  block_type=gatewayout
  sim_out_reg_sim_delay : xbsIndex_r4/Delay  rst=off  infoeditControl=Selection of Reset will increase slice count due to use of real FFs and instead of SRLs  en=off  latency=1  reg_retiming=on  dbl_ovrd=off  block_type=delay
  sim_out_reg : Outport
  wires:
  sim_out_reg_sim_delay/1 -> sim_out_reg_gw/1
  sim_out_reg_gw/1 -> sim_out_reg/1
  io_delay/1 -> cast_gw/1
  cast_gw/1 -> adm_pcie_9h7_dts_dual_4x100g_dsp_8b_1ant_pipeline_tt_offset_user_data_in/1
  adm_pcie_9h7_dts_dual_4x100g_dsp_8b_1ant_pipeline_tt_offset_user_data_in/1 -> sim_out/1
  out_reg/1 -> sim_out_reg_sim_delay/1, assert_reg/1
  assert_reg/1 -> reint1/1
  reint1/1 -> io_delay/1
